simulink model "control_lqr"  (R2025b)
settings: Solver=ode23t  StartTime=0.0  StopTime=10.0  MaxStep=1e-3  RelTol=1e-3  AbsTol=1e-3
undefined symbols (not defined in the file): K, Kf, p0
libraries: simulink_extras x2
settings Model: Creator=upattacini  LastModifiedBy=upattacini
settings DataIOCC: SaveOutput=off  DSMLogging=off  SaveTime=off
settings ModelReferenceCC: UpdateModelReferenceTargets=Force

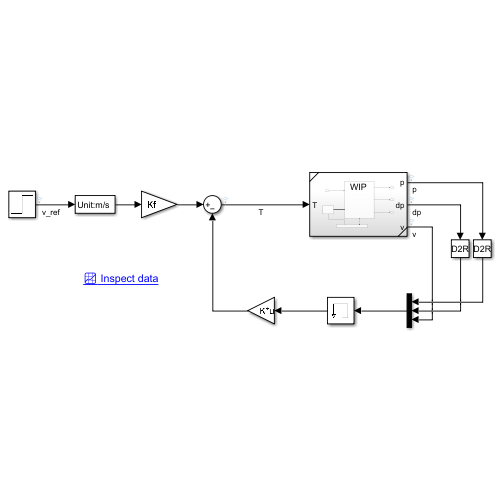
[thumbnail: Simulink's stored preview of the top-level diagram]
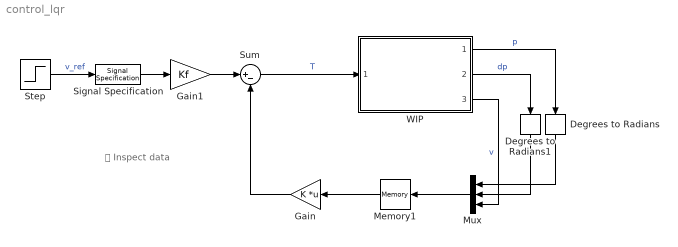
== system control_lqr ==
  note: 📈 Inspect data
  Degrees to Radians : simulink_extras/Transformations/Degrees to Radians
  Degrees to Radians1 : simulink_extras/Transformations/Degrees to Radians
  Gain : Gain  Gain=K  Multiplication=Matrix(K*u)
  Gain1 : Gain  Gain=Kf
  Memory1 : Memory  InitialCondition=[p0*pi/180 0 0]  InheritSampleTime=on  LinearizeMemory=on  LinearizeAsDelay=on
  Mux : Mux  Inputs=3
  Signal Specification : SignalSpecification  Unit=m/s
  Step : Step  SampleTime=0
  Sum : Sum  Inputs=|+-
  WIP : Subsystem  ReferencedSubsystem=WIP
  wires:
  Degrees to Radians/1 -> Mux/1
  WIP/2 -> Degrees to Radians1/1  "dp"
  Degrees to Radians1/1 -> Mux/2
  Gain1/1 -> Sum/1
  Memory1/1 -> Gain/1
  Gain/1 -> Sum/2
  WIP/3 -> Mux/3  "v"
  Mux/1 -> Memory1/1
  Step/1 -> Signal Specification/1  "v_ref"
  Signal Specification/1 -> Gain1/1
  Sum/1 -> WIP/1  "T"
  WIP/1 -> Degrees to Radians/1  "p"
